simulink model "c63_cylinder_combustion_ref"  (R2026a)
settings: Solver=ode4  StopTime=S12_CycleStopTimeS  FixedStep=1e-6
model workspace (MAT data in the model file):
  S12_C63_BoreM = Simulink.Parameter
  S12_C63_BoreM.Value = 0.1022
  S12_C63_BoreM.Complexity = 'real'
  S12_C63_BoreM.Dimensions = [1 1]
  S12_C63_BoreM.Description = 'Grade A: Mercedes-Benz Public Archive M156.985 bore'
  S12_C63_BoreM.DataType = 'auto'
  S12_C63_BoreM.DocUnits = 'm'
  S12_C63_CompressionRatio = Simulink.Parameter
  S12_C63_CompressionRatio.Value = 11.3
  S12_C63_CompressionRatio.Complexity = 'real'
  S12_C63_CompressionRatio.Dimensions = [1 1]
  S12_C63_CompressionRatio.Description = 'Grade A: Mercedes-Benz Public Archive M156.985 compression ratio'
  S12_C63_CompressionRatio.DataType = 'auto'
  S12_C63_RodLengthM = Simulink.Parameter
  S12_C63_RodLengthM.Value = 0.1455
  S12_C63_RodLengthM.Complexity = 'real'
  S12_C63_RodLengthM.Dimensions = [1 1]
  S12_C63_RodLengthM.Description = 'Grade D initial value; identify within 0.140 to 0.155 m'
  S12_C63_RodLengthM.DataType = 'auto'
  S12_C63_RodLengthM.DocUnits = 'm'
  S12_C63_StrokeM = Simulink.Parameter
  S12_C63_StrokeM.Value = 0.0946
  S12_C63_StrokeM.Complexity = 'real'
  S12_C63_StrokeM.Dimensions = [1 1]
  S12_C63_StrokeM.Description = 'Grade A: Mercedes-Benz Public Archive M156.985 stroke'
  S12_C63_StrokeM.DataType = 'auto'
  S12_C63_StrokeM.DocUnits = 'm'
  S12_CrankDegPerSecond = Simulink.Parameter
  S12_CrankDegPerSecond.Value = 18000
  S12_CrankDegPerSecond.Complexity = 'real'
  S12_CrankDegPerSecond.Dimensions = [1 1]
  S12_CrankDegPerSecond.Description = 'Derived crank angular speed'
  S12_CrankDegPerSecond.DataType = 'auto'
  S12_CrankDegPerSecond.DocUnits = 'deg/s'
  S12_CvJkgK = Simulink.Parameter
  S12_CvJkgK.Value = 718
  S12_CvJkgK.Complexity = 'real'
  S12_CvJkgK.Dimensions = [1 1]
  S12_CvJkgK.Description = 'Reference constant cv; replace with temperature table'
  S12_CvJkgK.DataType = 'auto'
  S12_CvJkgK.DocUnits = 'J/(kg*K)'
  S12_CycleStopTimeS = Simulink.Parameter
  S12_CycleStopTimeS.Value = 0.0172222222222
  S12_CycleStopTimeS.Complexity = 'real'
  S12_CycleStopTimeS.Dimensions = [1 1]
  S12_CycleStopTimeS.Description = 'Duration from -180 deg BDC to +130 deg ATDC'
  S12_CycleStopTimeS.DataType = 'auto'
  S12_CycleStopTimeS.DocUnits = 's'
  S12_EngineRPM = Simulink.Parameter
  S12_EngineRPM.Value = 3000
  S12_EngineRPM.Complexity = 'real'
  S12_EngineRPM.Dimensions = [1 1]
  S12_EngineRPM.Description = 'Reference operating point; not a fixed vehicle parameter'
  S12_EngineRPM.DataType = 'auto'
  S12_EngineRPM.DocUnits = 'rpm'
  S12_GasConstantJkgK = Simulink.Parameter
  S12_GasConstantJkgK.Value = 287
  S12_GasConstantJkgK.Complexity = 'real'
  S12_GasConstantJkgK.Dimensions = [1 1]
  S12_GasConstantJkgK.Description = 'Reference air value; replace with composition table'
  S12_GasConstantJkgK.DataType = 'auto'
  S12_GasConstantJkgK.DocUnits = 'J/(kg*K)'
  S12_HeatPerCycleJ = Simulink.Parameter
  S12_HeatPerCycleJ.Value = 2100
  S12_HeatPerCycleJ.Complexity = 'real'
  S12_HeatPerCycleJ.Dimensions = [1 1]
  S12_HeatPerCycleJ.Description = 'Grade D full-load chemical heat initial value; identify from IMEP'
  S12_HeatPerCycleJ.DataType = 'auto'
  S12_HeatPerCycleJ.DocUnits = 'J'
  S12_InitialPressurePa = Simulink.Parameter
  S12_InitialPressurePa.Value = 101325
  S12_InitialPressurePa.Complexity = 'real'
  S12_InitialPressurePa.Dimensions = [1 1]
  S12_InitialPressurePa.Description = 'Closed-cylinder reference initial pressure at BDC'
  S12_InitialPressurePa.DataType = 'auto'
  S12_InitialPressurePa.DocUnits = 'Pa'
  S12_InitialTemperatureK = Simulink.Parameter
  S12_InitialTemperatureK.Value = 330
  S12_InitialTemperatureK.Complexity = 'real'
  S12_InitialTemperatureK.Dimensions = [1 1]
  S12_InitialTemperatureK.Description = 'Closed-cylinder reference initial temperature at BDC'
  S12_InitialTemperatureK.DataType = 'auto'
  S12_InitialTemperatureK.DocUnits = 'K'
  S12_TrappedMassKg = Simulink.Parameter
  S12_TrappedMassKg.Value = 0.000910845682241
  S12_TrappedMassKg.Complexity = 'real'
  S12_TrappedMassKg.Dimensions = [1 1]
  S12_TrappedMassKg.Description = 'Derived BDC trapped mass from pV=mRT reference state'
  S12_TrappedMassKg.DataType = 'auto'
  S12_TrappedMassKg.DocUnits = 'kg'
  S12_WallTemperatureK = Simulink.Parameter
  S12_WallTemperatureK.Value = 430
  S12_WallTemperatureK.Complexity = 'real'
  S12_WallTemperatureK.Dimensions = [1 1]
  S12_WallTemperatureK.Description = 'Reference warm wall temperature'
  S12_WallTemperatureK.DataType = 'auto'
  S12_WallTemperatureK.DocUnits = 'K'
  S12_WiebeA = Simulink.Parameter
  S12_WiebeA.Value = 6.9
  S12_WiebeA.Complexity = 'real'
  S12_WiebeA.Dimensions = [1 1]
  S12_WiebeA.Description = 'Wiebe completion parameter from literature initialization'
  S12_WiebeA.DataType = 'auto'
  S12_WiebeDurationDeg = Simulink.Parameter
  S12_WiebeDurationDeg.Value = 50
  S12_WiebeDurationDeg.Complexity = 'real'
  S12_WiebeDurationDeg.Dimensions = [1 1]
  S12_WiebeDurationDeg.Description = 'Grade D combustion duration initial value'
  S12_WiebeDurationDeg.DataType = 'auto'
  S12_WiebeDurationDeg.DocUnits = 'deg'
  S12_WiebeM = Simulink.Parameter
  S12_WiebeM.Value = 2
  S12_WiebeM.Complexity = 'real'
  S12_WiebeM.Dimensions = [1 1]
  S12_WiebeM.Description = 'Grade D Wiebe shape initial value'
  S12_WiebeM.DataType = 'auto'
  S12_WiebeStartDeg = Simulink.Parameter
  S12_WiebeStartDeg.Value = -20
  S12_WiebeStartDeg.Complexity = 'real'
  S12_WiebeStartDeg.Dimensions = [1 1]
  S12_WiebeStartDeg.Description = 'Grade D combustion phasing initial value'
  S12_WiebeStartDeg.DataType = 'auto'
  S12_WiebeStartDeg.DocUnits = 'deg'
settings Model: Creator=Jovi  LastModifiedBy=Jovi

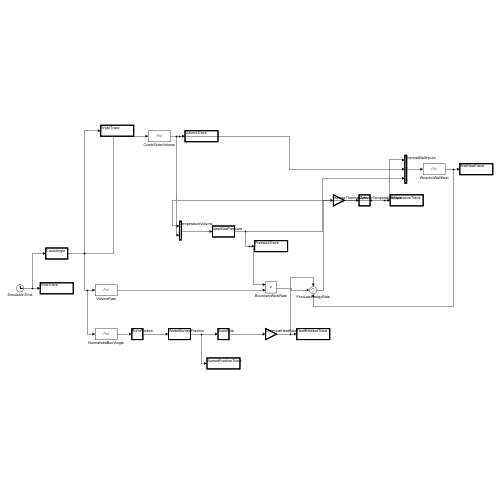
[thumbnail: Simulink's stored preview of the top-level diagram]
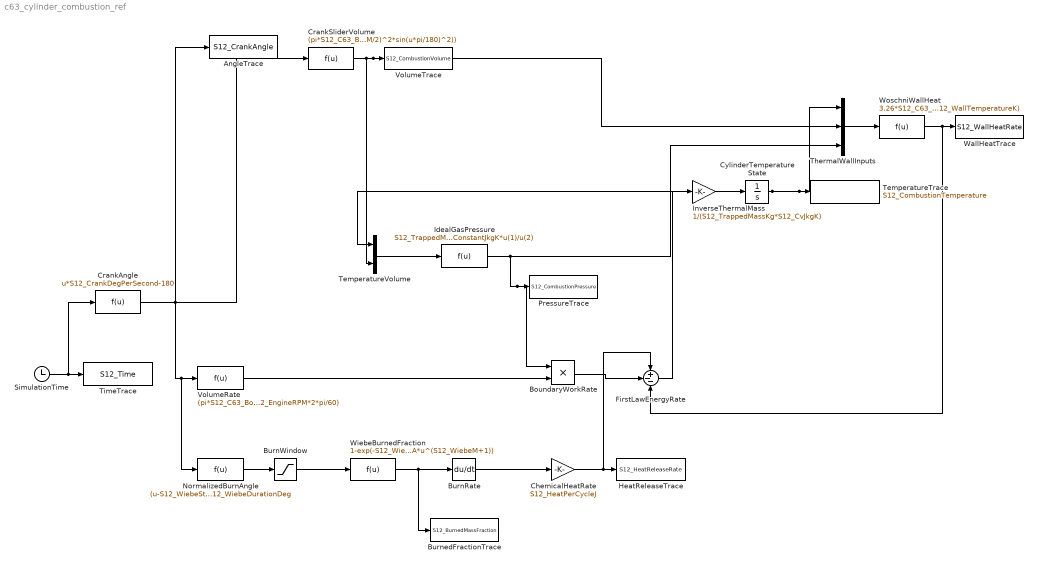
== system c63_cylinder_combustion_ref ==
  AngleTrace : ToWorkspace  VariableName=S12_CrankAngle
      settings: MaxDataPoints=50000
  BoundaryWorkRate : Product
  BurnRate : Derivative
  BurnWindow : Saturate  UpperLimit=1  LowerLimit=0
  BurnedFractionTrace : ToWorkspace  VariableName=S12_BurnedMassFraction
      settings: MaxDataPoints=50000
  ChemicalHeatRate : Gain  Gain=S12_HeatPerCycleJ
  CrankAngle : Fcn  Expr=u*S12_CrankDegPerSecond-180
  CrankSliderVolume : Fcn  Expr=(pi*S12_C63_BoreM^2*S12_C63_StrokeM/4)/(S12_C63_CompressionRatio-1)+(pi*S12_C63_BoreM^2/4)*((S12_C63_StrokeM/2)*(1-cos(u*pi/180))+S12_C63_RodLengthM-sqrt(S12_C63_RodLengthM^2-(S12_C63_StrokeM/2)^2*sin(u*pi/180)^2))
  CylinderTemperatureState : Integrator  InitialCondition=S12_InitialTemperatureK
  FirstLawEnergyRate : Sum  Inputs=+--
  HeatReleaseTrace : ToWorkspace  VariableName=S12_HeatReleaseRate
      settings: MaxDataPoints=50000
  IdealGasPressure : Fcn  Expr=S12_TrappedMassKg*S12_GasConstantJkgK*u(1)/u(2)
  InverseThermalMass : Gain  Gain=1/(S12_TrappedMassKg*S12_CvJkgK)
  NormalizedBurnAngle : Fcn  Expr=(u-S12_WiebeStartDeg)/S12_WiebeDurationDeg
  PressureTrace : ToWorkspace  VariableName=S12_CombustionPressure
      settings: MaxDataPoints=50000
  SimulationTime : Clock
  TemperatureTrace : ToWorkspace  VariableName=S12_CombustionTemperature
      settings: MaxDataPoints=50000
  TemperatureVolume : Mux  Inputs=2
  ThermalWallInputs : Mux  Inputs=3
  TimeTrace : ToWorkspace  VariableName=S12_Time
      settings: MaxDataPoints=50000
  VolumeRate : Fcn  Expr=(pi*S12_C63_BoreM^2/4)*((S12_C63_StrokeM/2)*sin(u*pi/180)+(S12_C63_StrokeM/2)^2*sin(u*pi/180)*cos(u*pi/180)/sqrt(S12_C63_RodLengthM^2-(S12_C63_StrokeM/2)^2*sin(u*pi/180)^2))*(S12_EngineRPM*2*pi/60)
  VolumeTrace : ToWorkspace  VariableName=S12_CombustionVolume
      settings: MaxDataPoints=50000
  WallHeatTrace : ToWorkspace  VariableName=S12_WallHeatRate
      settings: MaxDataPoints=50000
  WiebeBurnedFraction : Fcn  Expr=1-exp(-S12_WiebeA*u^(S12_WiebeM+1))
  WoschniWallHeat : Fcn  Expr=3.26*S12_C63_BoreM^(-0.2)*(u(3)/1000)^0.8*u(1)^(-0.55)*(2.28*(2*S12_C63_StrokeM*S12_EngineRPM/60))^0.8*(2*pi*S12_C63_BoreM^2/4+pi*S12_C63_BoreM*((u(2)-(pi*S12_C63_BoreM^2*S12_C63_StrokeM/4)/(S12_C63_CompressionRatio-1))/(pi*S12_C63_BoreM^2/4)))*(u(1)-S12_WallTemperatureK)
  wires:
  InverseThermalMass/1 -> CylinderTemperatureState/1
  FirstLawEnergyRate/1 -> InverseThermalMass/1
  WoschniWallHeat/1 -> FirstLawEnergyRate/3, WallHeatTrace/1
  ThermalWallInputs/1 -> WoschniWallHeat/1
  BoundaryWorkRate/1 -> FirstLawEnergyRate/2
  VolumeRate/1 -> BoundaryWorkRate/2
  IdealGasPressure/1 -> PressureTrace/1, BoundaryWorkRate/1, ThermalWallInputs/3
  TemperatureVolume/1 -> IdealGasPressure/1
  CylinderTemperatureState/1 -> ThermalWallInputs/1, TemperatureTrace/1, TemperatureVolume/1
  ChemicalHeatRate/1 -> FirstLawEnergyRate/1, HeatReleaseTrace/1
  BurnRate/1 -> ChemicalHeatRate/1
  WiebeBurnedFraction/1 -> BurnRate/1, BurnedFractionTrace/1
  CrankSliderVolume/1 -> ThermalWallInputs/2, VolumeTrace/1, TemperatureVolume/2
  CrankAngle/1 -> VolumeRate/1, NormalizedBurnAngle/1, AngleTrace/1, CrankSliderVolume/1
  SimulationTime/1 -> CrankAngle/1, TimeTrace/1
  NormalizedBurnAngle/1 -> BurnWindow/1
  BurnWindow/1 -> WiebeBurnedFraction/1
